simulink model "DSMC_params"  (R2021b)
settings: Solver=VariableStepDiscrete  StartTime=0.0  StopTime=30  FixedStep=0.02  MaxStep=Ts  RelTol=1e-3
PreLoadFcn:
  | if ~exist('sim_HIL')
  |     sim_HIL=false;
  | end
  | if ~exist('usefilter')
  |     usefilter=false;
  | end
InitFcn:
  | load motorModel.mat
  | load expsetup
model workspace (MAT data in the model file):
  Ts_path = 0.015
undefined symbols (not defined in the file): C, del, eta, gamm, k_lp, mModel, nodeID, qT, tau_lp, vphi, x28_000006_reduction, xiT
libraries: eeGeneralControl x1, dspsrcs4 x1, simulink x1
settings Model: DataDictionary=MotorInfo.sldd  SimulationMode=accelerator  SILPILSystemUnderTest=refmodels  Creator=khoi  LastModifiedBy=khoi
settings SolverCC: AlgebraicLoopSolver=TrustRegion
settings OptimizationCC: UseDivisionForNetSlopeComputation=on
settings DebuggingCC: AlgebraicLoopMsg=none  SFMachineParentedDataDiag=warning

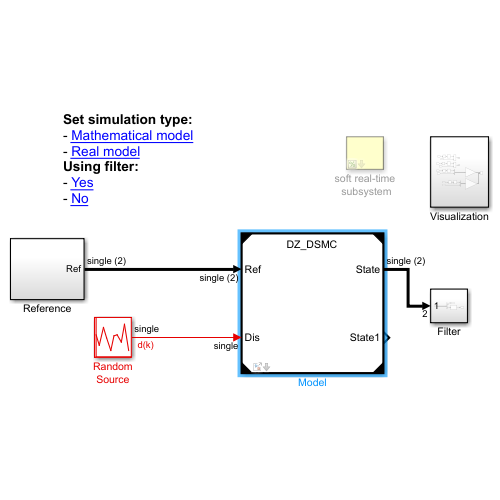
[thumbnail: Simulink's stored preview of the top-level diagram]
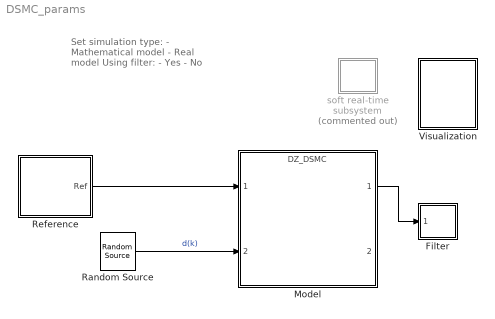
== system DSMC_params ==
  note: Set simulation type:
      | - Mathematical model
      | - Real model
      | Using filter:
      | - Yes
      | - No
  Filter : Subsystem
  Model : ModelReference  ModelNameDialog=DZ_DSMC.slx  UsingDefaultArgumentValue=0,0,0,0,0,0,0,0,0  ModelReferenceVersion=4.76  Phi=single(mModel{nodeID,3}.A)  Gam=single(mModel{nodeID,3}.B)  del=single(del)  eta=single(eta)  gamm=uint8(gamm)  qT=single(qT)  vphi=single(vphi)  xiT=single(xiT)  C=single(C)
  Random Source : dspsrcs4/Random Source  SrcType=Gaussian  NormMethod=Ziggurat  CltLength=12  MinVal=0  MaxVal=1  MeanVal=0  VarVal=1  RepMode=Not repeatable  rawSeed=1  IsInherit=off  SampMode=Discrete  SampTime=Ts  SampFrame=1  DataType=Single  OutComplex=Real  OutputFrames=off
  Reference : Subsystem
  Visualization : Subsystem
  soft real-time subsystem : Subsystem  Commented=on  mask{t_sample=0.01}
      mask prompts: t_sample "Sleep function interval (s)"
  wires:
  Random Source/1 -> Model/2  "d(k)"
  Model/1 -> Filter/1(Input)
  Reference/1(Ref) -> Model/1

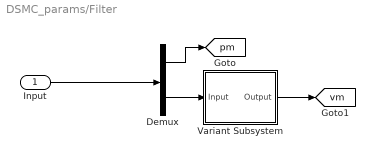
== system DSMC_params/Filter ==
  Input : Inport
  Demux : Demux  Outputs=2
  Variant Subsystem : Subsystem  Variant=on
  tag scope: pm=global, vm=global
  wires:
  Demux/2 -> Variant Subsystem/1(Input)
  Demux/1 -> [pm]
  Variant Subsystem/1(Output) -> [vm]
  Input/1 -> Demux/1

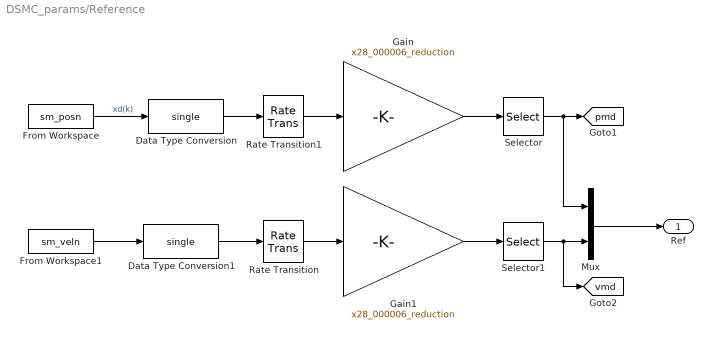
== system DSMC_params/Reference ==
  Data Type Conversion : DataTypeConversion  OutDataTypeStr=single
  Data Type Conversion1 : DataTypeConversion  OutDataTypeStr=single
  From Workspace : FromWorkspace  VariableName=sm_posn  SampleTime=Ts_path
  From Workspace1 : FromWorkspace  VariableName=sm_veln  SampleTime=Ts_path
  Gain : Gain  Gain=x28_000006_reduction  OutDataTypeStr=Inherit: Same as input
  Gain1 : Gain  Gain=x28_000006_reduction  OutDataTypeStr=Inherit: Same as input
  Mux : Mux  Inputs=2
  Rate Transition : RateTransition  OutPortSampleTime=Ts
  Rate Transition1 : RateTransition  OutPortSampleTime=Ts
  Selector : Selector  IndexMode=Zero-based  InputPortWidth=4  IndexOptions=Index vector (dialog)  Indices=nodeID-1  OutputSizes=1
  Selector1 : Selector  IndexMode=Zero-based  InputPortWidth=4  IndexOptions=Index vector (dialog)  Indices=nodeID-1  OutputSizes=1
  Ref : Outport
  tag scope: pmd=global, vmd=global
  wires:
  Mux/1 -> Ref/1
  Gain/1 -> Selector/1
  From Workspace/1 -> Data Type Conversion/1  "xd(k)"
  From Workspace1/1 -> Data Type Conversion1/1
  Gain1/1 -> Selector1/1
  Selector1/1 -> Mux/2, [vmd]
  Selector/1 -> Mux/1, [pmd]
  Rate Transition/1 -> Gain1/1
  Rate Transition1/1 -> Gain/1
  Data Type Conversion/1 -> Rate Transition1/1
  Data Type Conversion1/1 -> Rate Transition/1

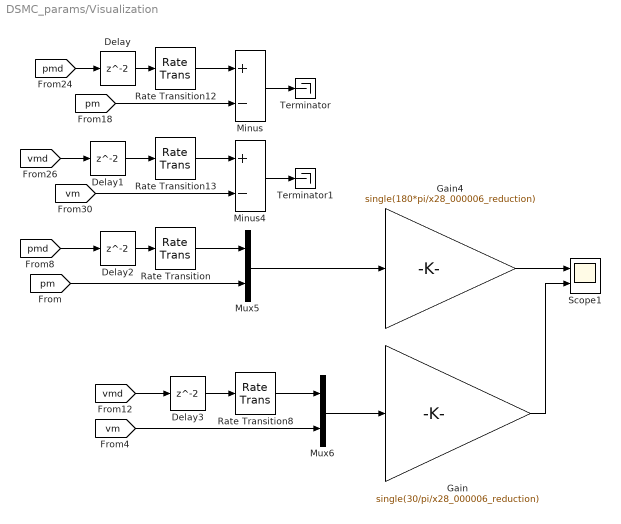
== system DSMC_params/Visualization ==
  Delay{,1..3} (4 alike) : Delay
  Gain : Gain  Gain=single(30/pi/x28_000006_reduction)
  Gain4 : Gain  Gain=single(180*pi/x28_000006_reduction)
  Minus : Sum  Inputs=+-
  Minus4 : Sum  Inputs=+-
  Mux5 : Mux  Inputs=2
  Mux6 : Mux  Inputs=2
  Rate Transition{,8,12..13} (4 alike) : RateTransition
  Scope1 : Scope  NumInputPorts=2
  Terminator : Terminator
  Terminator1 : Terminator
  wires:
  Rate Transition8/1 -> Mux6/1
  Rate Transition13/1 -> Minus4/1
  Mux5/1 -> Gain4/1
  Rate Transition12/1 -> Minus/1
  [vmd] -> Delay1/1
  [vmd] -> Delay3/1
  Gain4/1 -> Scope1/1
  Rate Transition/1 -> Mux5/1
  [pmd] -> Delay/1
  [pmd] -> Delay2/1
  Minus/1 -> Terminator/1
  Mux6/1 -> Gain/1
  Gain/1 -> Scope1/2
  Minus4/1 -> Terminator1/1
  [pm] -> Minus/2
  [vm] -> Minus4/2
  [pm] -> Mux5/2
  [vm] -> Mux6/2
  Delay3/1 -> Rate Transition8/1
  Delay2/1 -> Rate Transition/1
  Delay1/1 -> Rate Transition13/1
  Delay/1 -> Rate Transition12/1

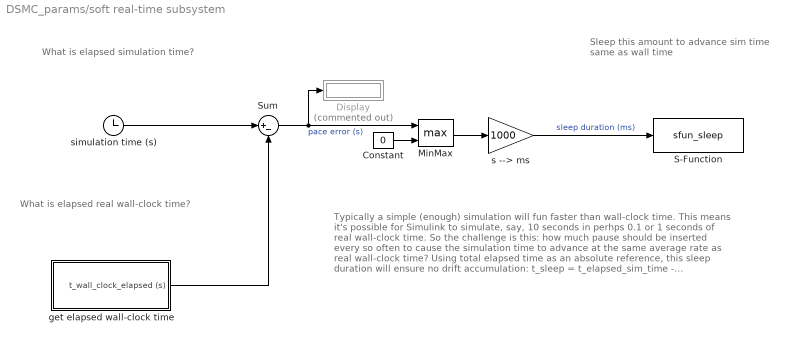
== system DSMC_params/soft real-time subsystem ==
  note: What is elapsed real
      | wall-clock time?
  note: What is elapsed
      | simulation time?
  note: Sleep this amount
      | to advance sim time
      | same as wall time
  note: Typically a simple (enough) simulation will fun faster than
      | wall-clock time. This means it's possible for Simulink to
      | simulate, say, 10 seconds in perhps 0.1 or 1 seconds of real
      | wall-clock time.
      |
      | So the challenge is this: how much pause should be inserted
      | every so often to cause the simulation time to advance at
      | the same average rate as real wall-clock time?
      |
      | Using total elapsed time as an absolute reference, this
      | sleep duration will ensure no drift accumulation:
      |
      | t_sleep = t_elapsed_sim_time - t_elapsed_wall_clock_time
      |
      | Pace error and Sleep() or usleep() resolution is system dependent
      | and likely around 10ms on Windows machines. Better on linux.
      |
      | Marc Compere
      | comperem@gmail.com
      | created : 28 May 2018
      | modified: 29 May 2018
      |
      | Reference:
      | Marc Compere (2022). S oft Real Time Block for Pacing Simulink Simulations (https://www.mathworks.com/matlabcentral/fileexchange/67520-soft-real-time-block-for-pacing-simulink-simulations), MATLAB Central File Exchange. Retrieved March 14, 2022.
  Constant : Constant  Value=0
  Display : Display  Commented=on
  MinMax : MinMax  Function=max  Inputs=2
  S-Function : S-Function  FunctionName=sfun_sleep  Parameters=t_sample  SFunctionDeploymentMode=off  EnableBusSupport=off
  Sum : Sum  Inputs=|+-
  get elapsed wall-clock time : Subsystem
  s --> ms : Gain  Gain=1000
  simulation time (s) : Clock
  wires:
  simulation time (s)/1 -> Sum/1
  Constant/1 -> MinMax/2
  get elapsed wall-clock time/1(t_wall_clock_elapsed (s)) -> Sum/2
  Sum/1 -> Display/1, MinMax/1  "pace error (s)"
  MinMax/1 -> s --> ms/1
  s --> ms/1 -> S-Function/1  "sleep duration (ms)"

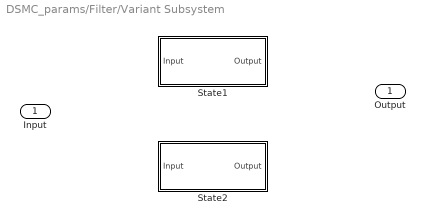
== system DSMC_params/Filter/Variant Subsystem ==
  Input : Inport
  State1 : Subsystem  VariantControl=usefilter == true
  State2 : Subsystem  VariantControl=usefilter == false
  Output : Outport

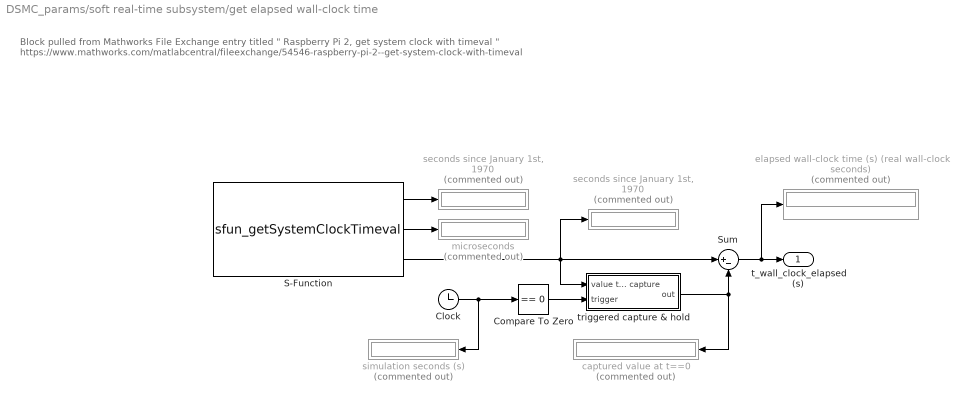
== system DSMC_params/soft real-time subsystem/get elapsed wall-clock time ==
  note: Block pulled from Mathworks File Exchange entry titled " Raspberry Pi 2, get system clock with timeval "
      |
      | https://www.mathworks.com/matlabcentral/fileexchange/54546-raspberry-pi-2--get-system-clock-with-timeval
  Clock : Clock
  Compare To Zero : simulink/Logic and Bit Operations/Compare To Zero  relop===  OutDataTypeStr=boolean
  S-Function : S-Function  FunctionName=sfun_getSystemClockTimeval  SFunctionDeploymentMode=off  EnableBusSupport=off
  Sum : Sum  Inputs=|+-
  captured value at t==0 : Display  Commented=on
  elapsed wall-clock time (s) (real wall-clock seconds) : Display  Commented=on
  microseconds : Display  Commented=on
  "seconds since January 1st, 1970" : Display  Commented=on
  "seconds since January 1st, 1970 " : Display  Commented=on
  simulation seconds (s) : Display  Commented=on
  triggered capture & hold : Subsystem
  t_wall_clock_elapsed (s) : Outport
  wires:
  triggered capture & hold/1(out) -> captured value at t==0/1, Sum/2
  S-Function/1 -> "seconds since January 1st, 1970 "/1
  Compare To Zero/1 -> triggered capture & hold/2(trigger)
  Sum/1 -> t_wall_clock_elapsed (s)/1, elapsed wall-clock time (s) (real wall-clock seconds)/1
  S-Function/2 -> microseconds/1
  S-Function/3 -> triggered capture & hold/1(value to capture), Sum/1, "seconds since January 1st, 1970"/1
  Clock/1 -> Compare To Zero/1, simulation seconds (s)/1

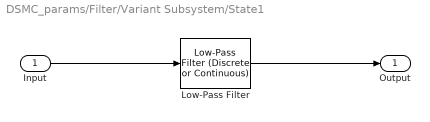
== system DSMC_params/Filter/Variant Subsystem/State1 ==
  Input : Inport
  Low-Pass Filter : eeGeneralControl/Low-Pass Filter (Discrete or Continuous)  K=k_lp(1)  T=tau_lp(1)  B=inf  A=-inf  init_option=Inherited from block input  x0=0  Ts=-1
  Output : Outport
  wires:
  Input/1 -> Low-Pass Filter/1
  Low-Pass Filter/1 -> Output/1

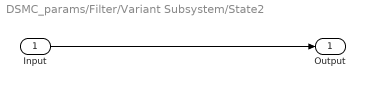
== system DSMC_params/Filter/Variant Subsystem/State2 ==
  Input : Inport
  Output : Outport
  wires:
  Input/1 -> Output/1

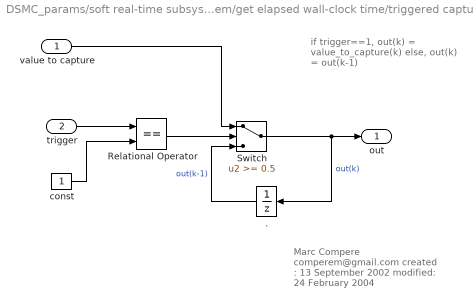
== system DSMC_params/soft real-time subsystem/get elapsed wall-clock time/triggered capture & hold ==
  note: Marc Compere
      | comperem@gmail.com
      | created  : 13 September 2002
      | modified: 24 February 2004
  note: if trigger==1,
      |    out(k) = value_to_capture(k)
      | else,
      |    out(k) = out(k-1)
  value to capture : Inport
  trigger : Inport  Port=2
  . : UnitDelay  SampleTime=-1  HasFrameUpgradeWarning=on
  Relational Operator : RelationalOperator  Operator===  RndMeth=Nearest
  Switch : Switch  Threshold=0.5  SaturateOnIntegerOverflow=on
  const : Constant
  out : Outport
  wires:
  trigger/1 -> Relational Operator/1
  const/1 -> Relational Operator/2
  Relational Operator/1 -> Switch/2
  Switch/1 -> ./1, out/1  "out(k)"
  value to capture/1 -> Switch/1
  ./1 -> Switch/3  "out(k-1)"
